simulink model "fermentation_dynamic_model"  (R2017b)
settings: Solver=VariableStepAuto  StartTime=0.0  StopTime=250  RelTol=1e-3
values from neighbouring files (symbols this model uses):
  E_0 = 0    [fermentation_config.m]    (also in fermentation_config_update.m)
  G_0 = 70    [fermentation_config.m]    (also in fermentation_config_update.m = 104.992339972)
  M_0 = 40    [fermentation_config.m]    (also in fermentation_config_update.m = 60)
  N_0 = 230    [fermentation_config.m]    (also in fermentation_config_update.m = 343.376857703)
  p_KG = polyfit(T,K_G,1)    [fermentation_config.m]    (also in fermentation_config_update.m)
  p_KiG = polyfit(T,Ki_G,1)    [fermentation_config.m]    (also in fermentation_config_update.m)
  p_KiM = polyfit(T,Ki_M,1)    [fermentation_config.m]    (also in fermentation_config_update.m)
  p_KM = polyfit(T,K_M,1)    [fermentation_config.m]    (also in fermentation_config_update.m)
  p_KN = polyfit(T,K_N,1)    [fermentation_config.m]    (also in fermentation_config_update.m)
  p_VG = polyfit(T,V_G,1)    [fermentation_config.m]    (also in fermentation_config_update.m)
  p_VM = polyfit(T,V_M,1)    [fermentation_config.m]    (also in fermentation_config_update.m)
  p_VN = polyfit(T,V_N,1)    [fermentation_config.m]    (also in fermentation_config_update.m)
  R_EG = 1.92    [fermentation_config.m]    (also in fermentation_config_update.m)
  R_EM = 3.84    [fermentation_config.m]    (also in fermentation_config_update.m)
  R_EN = 5.76    [fermentation_config.m]    (also in fermentation_config_update.m)
  R_XG = 0.134    [fermentation_config.m]    (also in fermentation_config_update.m)
  R_XM = 0.268    [fermentation_config.m]    (also in fermentation_config_update.m)
  R_XN = 0.402    [fermentation_config.m]    (also in fermentation_config_update.m)
  T_c = 2    [fermentation_config.m]    (also in fermentation_config_update.m = 12)
  T_s = 15    [fermentation_config.m]    (also in fermentation_config_update.m = 12)
  X_0 = 200    [fermentation_config.m]    (also in fermentation_config_update.m)
settings Model: Creator=Alexander  LastModifiedBy=Alexander

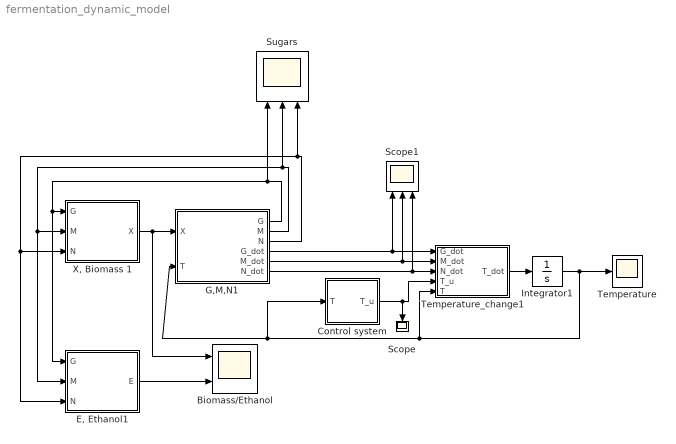
== system fermentation_dynamic_model ==
  Biomass/Ethanol : Scope  NumInputPorts=2
  Control system : Subsystem
  "E, Ethanol1" : Subsystem
  G,M,N1 : Subsystem
  Integrator1 : Integrator  InitialCondition=2
  Scope : Scope
  Scope1 : Scope  NumInputPorts=3
  Sugars : Scope  NumInputPorts=3
  Temperature : Scope
  Temperature_change1 : MATLAB Function  TreatAsAtomicUnit=on
  "X, Biomass 1" : Subsystem
  wires:
  G,M,N1/4(G_dot) -> Scope1/1, Temperature_change1/1(G_dot)
  G,M,N1/3(N) -> "X, Biomass 1"/3(N), "E, Ethanol1"/3(N), Sugars/3
  "E, Ethanol1"/1(E) -> Biomass/Ethanol/2
  "X, Biomass 1"/1(X) -> Biomass/Ethanol/1, G,M,N1/1(X)
  G,M,N1/2(M) -> "E, Ethanol1"/2(M), "X, Biomass 1"/2(M), Sugars/2
  Integrator1/1 -> Temperature/1, Control system/1(T), G,M,N1/2("T "), Temperature_change1/5(T)
  G,M,N1/6(N_dot) -> Scope1/3, Temperature_change1/3(N_dot)
  G,M,N1/5(M_dot) -> Scope1/2, Temperature_change1/2(M_dot)
  Temperature_change1/1(T_dot) -> Integrator1/1
  Control system/1(T_u) -> Scope/1, Temperature_change1/4(T_u)
  G,M,N1/1(G) -> "E, Ethanol1"/1(G), "X, Biomass 1"/1(G), Sugars/1

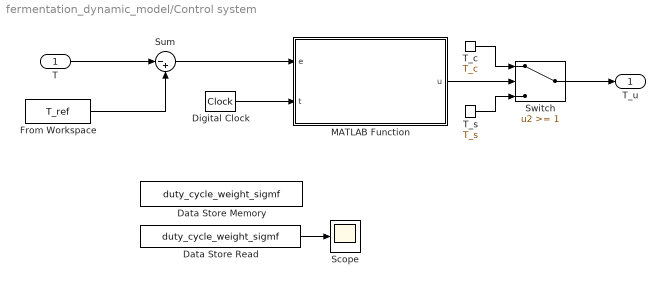
== system fermentation_dynamic_model/Control system ==
  T : Inport
  Data Store Memory : DataStoreMemory  DataStoreName=duty_cycle_weight_sigmf  ReadBeforeWriteMsg=warning  WriteAfterWriteMsg=warning  WriteAfterReadMsg=warning  ShowAdditionalParam=off  OutDataTypeStr=double
  Data Store Read : DataStoreRead  DataStoreName=duty_cycle_weight_sigmf
  Digital Clock : DigitalClock  SampleTime=0.01
  From Workspace : FromWorkspace  VariableName=T_ref  SampleTime=0
  MATLAB Function : MATLAB Function  TreatAsAtomicUnit=on
  Scope : Scope
  Sum : Sum  Inputs=|-+
  Switch : Switch  Threshold=1
  T_c : Constant  Value=T_c
  T_s : Constant  Value=T_s
  T_u : Outport
  wires:
  T/1 -> Sum/1
  Sum/1 -> MATLAB Function/1(e)
  MATLAB Function/1(u) -> Switch/2
  T_c/1 -> Switch/1
  T_s/1 -> Switch/3
  Switch/1 -> T_u/1
  Digital Clock/1 -> MATLAB Function/2(t)
  From Workspace/1 -> Sum/2
  Data Store Read/1 -> Scope/1

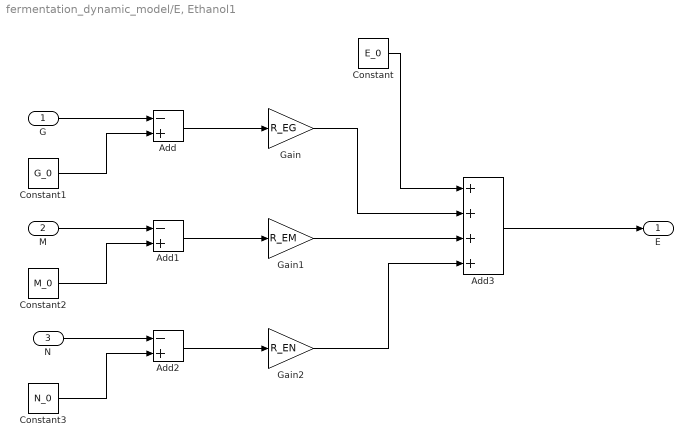
== system fermentation_dynamic_model/E, Ethanol1 ==
  G : Inport
  M : Inport  Port=2
  N : Inport  Port=3
  Add : Sum  Inputs=-+
  Add1 : Sum  Inputs=-+
  Add2 : Sum  Inputs=-+
  Add3 : Sum  Inputs=++++
  Constant : Constant  Value=E_0
  Constant1 : Constant  Value=G_0
  Constant2 : Constant  Value=M_0
  Constant3 : Constant  Value=N_0
  Gain : Gain  Gain=R_EG
  Gain1 : Gain  Gain=R_EM
  Gain2 : Gain  Gain=R_EN
  E : Outport
  wires:
  G/1 -> Add/1
  M/1 -> Add1/1
  N/1 -> Add2/1
  Constant3/1 -> Add2/2
  Constant2/1 -> Add1/2
  Constant1/1 -> Add/2
  Add/1 -> Gain/1
  Add1/1 -> Gain1/1
  Add2/1 -> Gain2/1
  Add3/1 -> E/1
  Constant/1 -> Add3/1
  Gain/1 -> Add3/2
  Gain1/1 -> Add3/3
  Gain2/1 -> Add3/4

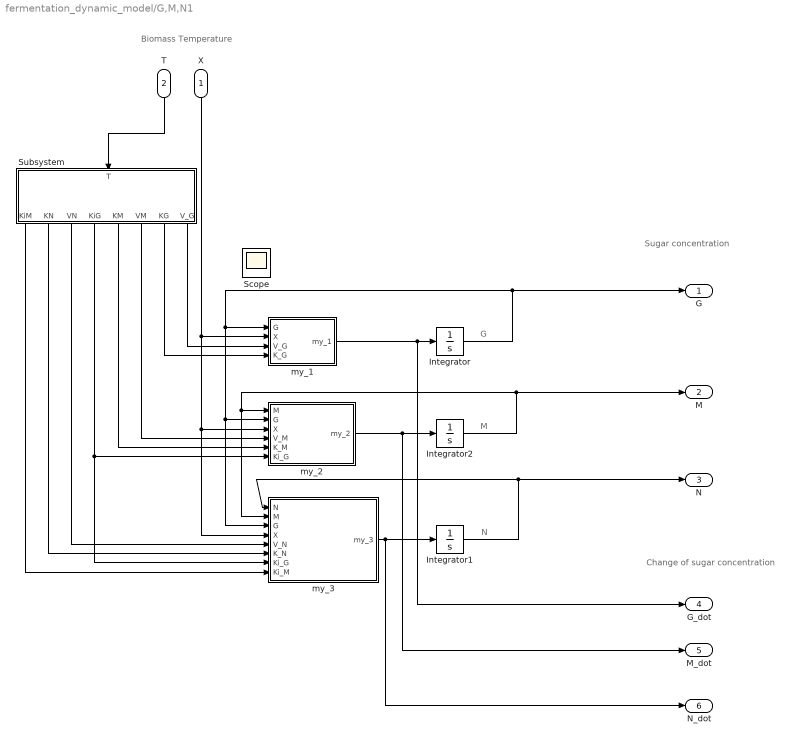
== system fermentation_dynamic_model/G,M,N1 ==
  note: Change of sugar
      | concentration
  note: Sugar concentration
  note: Biomass
      | Temperature
  note: N
  note: M
  note: G
  X : Inport
  "T " : Inport  Port=2
  Integrator : Integrator  InitialCondition=G_0
  Integrator1 : Integrator  InitialCondition=N_0
  Integrator2 : Integrator  InitialCondition=M_0
  Scope : Scope  NumInputPorts=3
  Subsystem : Subsystem
  my_1 : MATLAB Function  TreatAsAtomicUnit=on
  my_2 : MATLAB Function  TreatAsAtomicUnit=on
  my_3 : MATLAB Function  TreatAsAtomicUnit=on
  G : Outport
  M : Outport  Port=2
  N : Outport  Port=3
  G_dot : Outport  Port=4
  M_dot : Outport  Port=5
  N_dot : Outport  Port=6
  wires:
  my_1/1(my_1) -> G_dot/1, Integrator/1
  Integrator/1 -> G/1, my_1/1(G), my_2/2(G), my_3/3(G)
  my_2/1(my_2) -> M_dot/1, Integrator2/1
  Integrator1/1 -> my_3/1(N), N/1
  Integrator2/1 -> my_3/2(M), my_2/1(M), M/1
  my_3/1(my_3) -> Integrator1/1, N_dot/1
  X/1 -> my_3/4(X), my_2/3(X), my_1/2(X)
  "T "/1 -> Subsystem/1(T)
  Subsystem/1(KiM) -> my_3/8(Ki_M)
  Subsystem/4(KiG) -> my_2/6(Ki_G), my_3/7(Ki_G)
  Subsystem/2(KN) -> my_3/6(K_N)
  Subsystem/3(VN) -> my_3/5(V_N)
  Subsystem/5(KM) -> my_2/5(K_M)
  Subsystem/6(VM) -> my_2/4(V_M)
  Subsystem/7(KG) -> my_1/4(K_G)
  Subsystem/8(V_G) -> my_1/3(V_G)

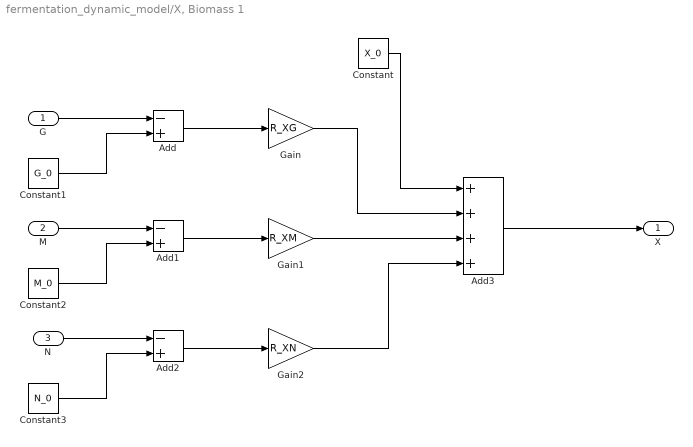
== system fermentation_dynamic_model/X, Biomass 1 ==
  G : Inport
  M : Inport  Port=2
  N : Inport  Port=3
  Add : Sum  Inputs=-+
  Add1 : Sum  Inputs=-+
  Add2 : Sum  Inputs=-+
  Add3 : Sum  Inputs=++++
  Constant : Constant  Value=X_0
  Constant1 : Constant  Value=G_0
  Constant2 : Constant  Value=M_0
  Constant3 : Constant  Value=N_0
  Gain : Gain  Gain=R_XG
  Gain1 : Gain  Gain=R_XM
  Gain2 : Gain  Gain=R_XN
  X : Outport
  wires:
  G/1 -> Add/1
  M/1 -> Add1/1
  N/1 -> Add2/1
  Constant3/1 -> Add2/2
  Constant2/1 -> Add1/2
  Constant1/1 -> Add/2
  Add/1 -> Gain/1
  Add1/1 -> Gain1/1
  Add2/1 -> Gain2/1
  Add3/1 -> X/1
  Constant/1 -> Add3/1
  Gain/1 -> Add3/2
  Gain1/1 -> Add3/3
  Gain2/1 -> Add3/4

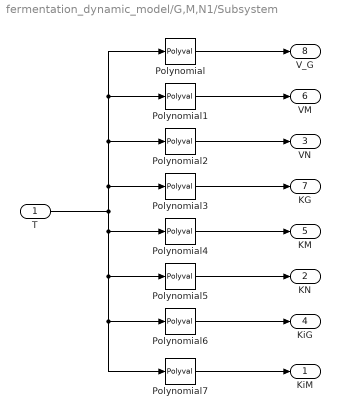
== system fermentation_dynamic_model/G,M,N1/Subsystem ==
  T : Inport
  Polynomial : Polyval  Coefs=p_VG
  Polynomial1 : Polyval  Coefs=p_VM
  Polynomial2 : Polyval  Coefs=p_VN
  Polynomial3 : Polyval  Coefs=p_KG
  Polynomial4 : Polyval  Coefs=p_KM
  Polynomial5 : Polyval  Coefs=p_KN
  Polynomial6 : Polyval  Coefs=p_KiG
  Polynomial7 : Polyval  Coefs=p_KiM
  KiM : Outport
  KN : Outport  Port=2
  VN : Outport  Port=3
  KiG : Outport  Port=4
  KM : Outport  Port=5
  VM : Outport  Port=6
  KG : Outport  Port=7
  V_G : Outport  Port=8
  wires:
  Polynomial/1 -> V_G/1
  Polynomial1/1 -> VM/1
  Polynomial2/1 -> VN/1
  Polynomial3/1 -> KG/1
  Polynomial4/1 -> KM/1
  Polynomial5/1 -> KN/1
  Polynomial6/1 -> KiG/1
  Polynomial7/1 -> KiM/1
  T/1 -> Polynomial2/1, Polynomial1/1, Polynomial/1, Polynomial3/1, Polynomial4/1, Polynomial7/1, Polynomial6/1, Polynomial5/1

== matlab function fermentation_dynamic_model/Control system/MATLAB Function ==
  settings: updateMethod=DISCRETE
  data: e input; u output; t input; duty_cycle_weight_sigmf data_store_memory
function u  = duty_cycle(e,t)
global  duty_cycle_weight_sigmf
% Slope of the sigmoid function
sig_slope = 3;
% Point of 1/2 output from the sigmoid function
sig_half= 0.23; 
% Duty time which gets divided to an active and an inactive phase
duty_cycle_time = 0.5;
% The modulus of the current time of the cycle time corresponds to
% percentage of the current cycle
t_in_cycle=mod(t,duty_cycle_time);

% Approx steady state active phase
if t_in_cycle ==0
duty_cycle_weight_sigmf = sigmf(e,[sig_slope,sig_half]);
end

if  t_in_cycle/duty_cycle_time > duty_cycle_weight_sigmf
    u=1;
else
    u=0;
end

== matlab function fermentation_dynamic_model/G,M,N1/my_1 ==
  data: G input; my_1 output; X input; V_G input; K_G input
function my_1 = fcn(G,X, V_G, K_G)
%#codegen

my_1 = -(V_G*G)/(K_G + G)*X;

== matlab function fermentation_dynamic_model/G,M,N1/my_2 ==
  data: M input; G input; my_2 output; X input; V_M input; K_M input; Ki_G input
function my_2 = fcn(M,G,X, V_M, K_M, Ki_G)
%#codegen

my_2 = -((V_M*M)/(K_M + M)*(Ki_G/(Ki_G + G)))*X;

== matlab function fermentation_dynamic_model/G,M,N1/my_3 ==
  data: N input; M input; G input; my_3 output; X input; V_N input; K_N input; Ki_G input; Ki_M input
function my_3 = fcn(N,M,G,X, V_N, K_N, Ki_G, Ki_M)
%#codegen



my_3 = -((V_N*N)/(K_N + N)*Ki_M/(Ki_M + M)*Ki_G/(Ki_G + G))*X;

== matlab function fermentation_dynamic_model/Temperature_change1 ==
  data: G_dot input; T_dot output; M_dot input; N_dot input; T_u input; T input
function T_dot = fcn(G_dot,M_dot,N_dot,T_u,T)
%#codegen

rho = 1.06;
Cp = 4000;

DH_RG = -91.2;
DH_RM = -226.3;
DH_RN = -361.3;

U = 1300;
Area = 0.188;
V = 1;

u = (U*Area)/V;

T_dot = 1/(rho*Cp)*(DH_RG*G_dot + DH_RM*M_dot + DH_RN*N_dot - u*(T - T_u));
